simulink model "Encoder"  (R2026a)
settings: Solver=FixedStepDiscrete  StopTime=inf  FixedStep=0.001
undefined symbols (not defined in the file or in its folder): Blocking, Non
libraries: amg_usbconverter_n_connect_lib x2
settings Model: Creator=pboon  LastModifiedBy=Admin

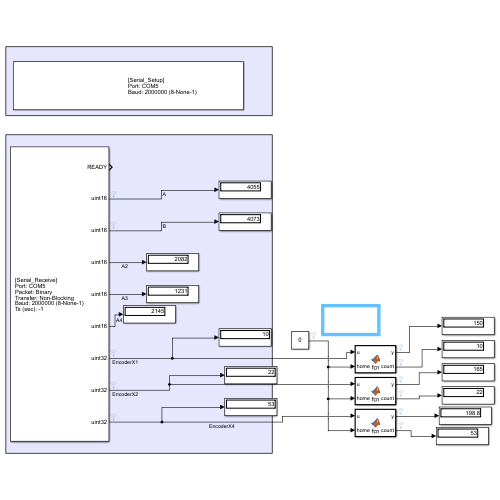
[thumbnail: Simulink's stored preview of the top-level diagram]
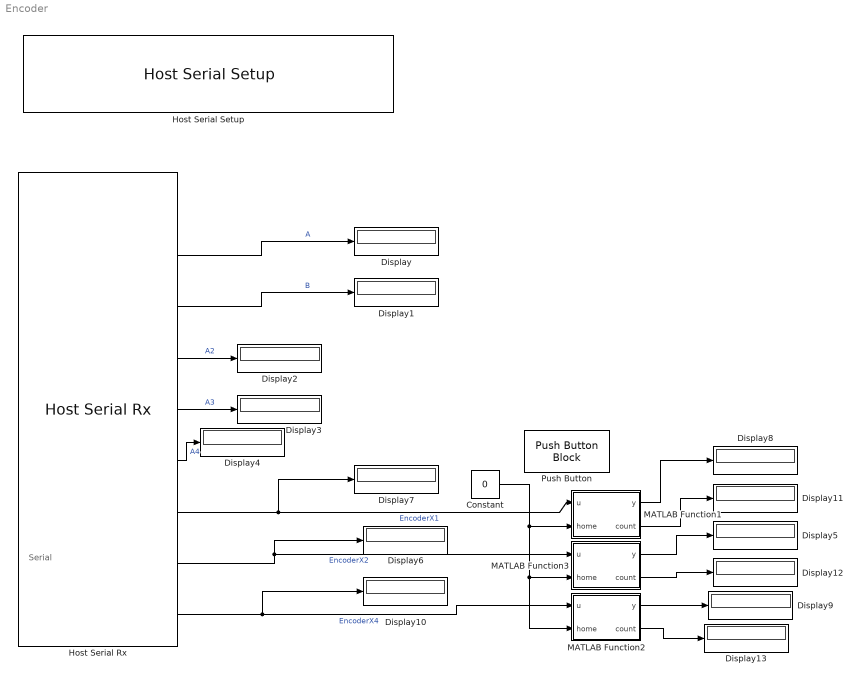
== system Encoder ==
  note: Serial
  Constant : Constant  Value=0
  Display{,1..13} (14 alike) : Display
  Host Serial Rx : amg_usbconverter_n_connect_lib/Host Serial Rx  conf=rx  port=<auto>  baudrate=2000000  databits=8  parity=None  stopbit=1  flowcontrol=None  transfer=Non-Blocking  timeout=5  packetmode=Binary  enableinitialvalues=off  initialvalues=[]  binheader='25'  binterminator='4E 4E'  porttype_double=0  porttype_single=0  porttype_int8=0  porttype_uint8=0  porttype_int16=0  porttype_uint16=5  porttype_int32=0  porttype_uint32=3  asciiformat='%d,%f'  rx_asciiterminator="CRLF (0x0D 0x0A - \"\\r\\n\")"  tx_asciiterminator="CRLF (0x0D 0x0A - \"\\r\\n\")"  sampletime=0.001  enablecustomportlabel=off  cinputportlabel=0  coutputportlabel=A  portpinstr=0  blockid=HostSerialRx  inputporttype=[]  inputportwidth=[]  inputportlabel={}  outputporttype=[3 5 5 5 5 5 7 7 7]  outputportwidth=[1 1 1 1 1 1 1 1 1]  outputportlabel={'READY','uint16','uint16','uint16','uint16','uint16','uint32','uint32','uint32'}  compat=0  optionstring=[]  autoport='COM5'
  Host Serial Setup : amg_usbconverter_n_connect_lib/Host Serial Setup  conf=setup  port=<auto>  baudrate=2000000  databits=8  parity=None  stopbit=1  flowcontrol=None  transfer=Blocking  timeout=2  packetmode=Binary  initialvalues=[]  binheader='7E 7E'  binterminator='03 03'  porttype_double=0  porttype_single=1  porttype_int8=0  porttype_uint8=0  porttype_int16=0  porttype_uint16=0  porttype_int32=0  porttype_uint32=2  asciiformat='%d %u %x'  rx_asciiterminator="CRLF (0x0D 0x0A - \"\\r\\n\")"  tx_asciiterminator="CRLF (0x0D 0x0A - \"\\r\\n\")"  sampletime=-1  enablecustomportlabel=off  cinputportlabel=0  coutputportlabel=A  portpinstr=0  blockid=HostSerialSetup  inputporttype=[]  inputportwidth=[]  inputportlabel={}  outputporttype=[]  outputportwidth=[]  outputportlabel={}  compat=0  optionstring=[]  autoport='COM5'
  MATLAB Function1 : MATLAB Function  TreatAsAtomicUnit=on
  MATLAB Function2 : MATLAB Function  TreatAsAtomicUnit=on
  MATLAB Function3 : MATLAB Function  TreatAsAtomicUnit=on
  Push Button : PushButtonBlock  IconOnColor=[0.0, 0.39215686274509803, 0.0]  IconOffColor=[0.0, 1.0, 0.0]  OffValue=0.000000
  wires:
  Host Serial Rx/2 -> Display/1  "A"
  Host Serial Rx/3 -> Display1/1  "B"
  Host Serial Rx/4 -> Display2/1  "A2"
  Host Serial Rx/5 -> Display3/1  "A3"
  Host Serial Rx/6 -> Display4/1  "A4"
  Host Serial Rx/8 -> MATLAB Function3/1(u), Display6/1  "EncoderX2"
  Host Serial Rx/9 -> MATLAB Function2/1(u), Display10/1  "EncoderX4"
  Host Serial Rx/7 -> MATLAB Function1/1(u), Display7/1  "EncoderX1"
  MATLAB Function1/1(y) -> Display8/1
  MATLAB Function2/1(y) -> Display9/1
  MATLAB Function3/1(y) -> Display5/1
  Constant/1 -> MATLAB Function2/2(home), MATLAB Function3/2(home), MATLAB Function1/2(home)
  MATLAB Function1/2(count) -> Display11/1
  MATLAB Function3/2(count) -> Display12/1
  MATLAB Function2/2(count) -> Display13/1

== matlab function Encoder/MATLAB Function3 ==
  data: u input; y output; home input; count output
function [y,count]= fcn(u, home)
persistent prev pos lastHome
c = double(u);

if isempty(prev)
    prev = c;
    pos = 0;
    lastHome = false;
end

d = c - prev;
if d > 32768
    d = d - 65536;
elseif d < -32768
    d = d + 65536;
end

pos = pos + d;
prev = c;

% ตั้งศูนย์เฉพาะจังหวะกดปุ่ม
pressed = (home ~= 0);
if pressed && ~lastHome
    pos = 0;
end
lastHome = pressed;
count = pos;
N = 48; % X1=24 2048, X2=48 4096, X4=96 8192
y = mod(pos, N) * (360/N);
end

== matlab function Encoder/MATLAB Function2 ==
  data: u input; y output; home input; count output
function [y,count]= fcn(u, home)
persistent prev pos lastHome
c = double(u);

if isempty(prev)
    prev = c;
    pos = 0;
    lastHome = false;
end

d = c - prev;
if d > 32768
    d = d - 65536;
elseif d < -32768
    d = d + 65536;
end

pos = pos + d;
prev = c;

% ตั้งศูนย์เฉพาะจังหวะกดปุ่ม
pressed = (home ~= 0);
if pressed && ~lastHome
    pos = 0;
end
lastHome = pressed;
count = pos;
N = 96; % X1=24 2048, X2=48 4096, X4=96 8192
y = mod(pos, N) * (360/N);
end

== matlab function Encoder/MATLAB Function1 ==
  data: u input; y output; home input; count output
function [y,count]= fcn(u, home)
persistent prev pos lastHome
c = double(u);

if isempty(prev)
    prev = c;
    pos = 0;
    lastHome = false;
end

d = c - prev;
if d > 32768
    d = d - 65536;
elseif d < -32768
    d = d + 65536;
end

pos = pos + d;
prev = c;

% ตั้งศูนย์เฉพาะจังหวะกดปุ่ม
pressed = (home ~= 0);
if pressed && ~lastHome
    pos = 0;
end
lastHome = pressed;
count = pos;
N = 24; % % X1=24 2048, X2=48 4096, X4=96 8192
y = mod(pos, N) * (360/N);
end
